simulink subsystem "Shaftline"  (R2024b)
settings: Solver=VariableStepAuto  StartTime=0.0  StopTime=10.0  RelTol=1e-3
undefined symbols (not defined in the file or in its folder): shaft
settings Model: Creator=Santiago  LastModifiedBy=Santiago

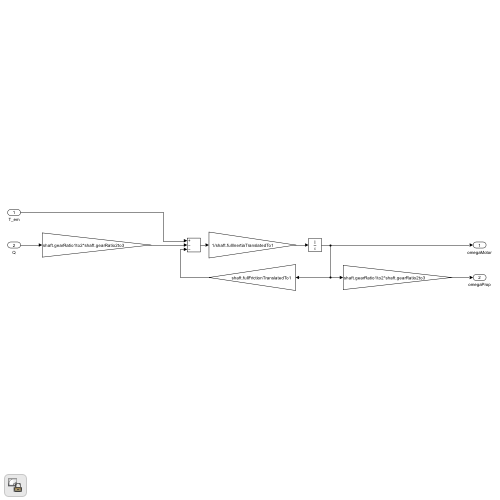
[thumbnail: Simulink's stored preview of the top-level diagram]
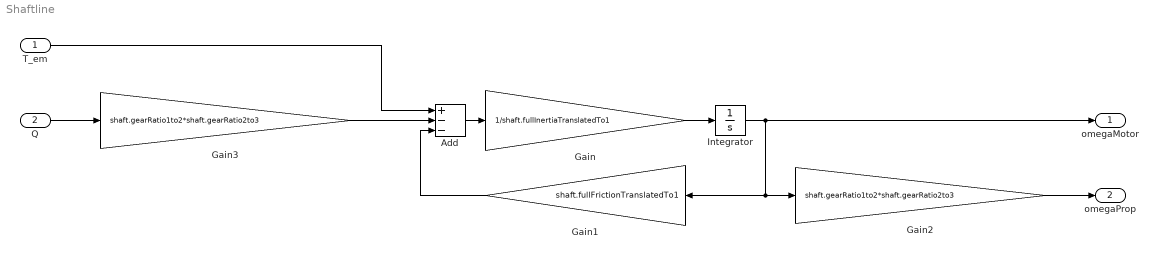
== system Shaftline ==
  T_em : Inport
  Q : Inport  Port=2
  Add : Sum  Inputs=+--
  Gain : Gain  Gain=1/shaft.fullInertiaTranslatedTo1
  Gain1 : Gain  Gain=shaft.fullFrictionTranslatedTo1
  Gain2 : Gain  Gain=shaft.gearRatio1to2*shaft.gearRatio2to3
  Gain3 : Gain  Gain=shaft.gearRatio1to2*shaft.gearRatio2to3
  Integrator : Integrator
  omegaMotor : Outport
  omegaProp : Outport  Port=2
  wires:
  Gain/1 -> Integrator/1
  Add/1 -> Gain/1
  Integrator/1 -> omegaMotor/1, Gain1/1, Gain2/1
  Gain1/1 -> Add/3
  T_em/1 -> Add/1
  Q/1 -> Gain3/1
  Gain2/1 -> omegaProp/1
  Gain3/1 -> Add/2
